simulink model "AEB_RuleBased_decisionmaking"  (R2021b)
settings: Solver=ode4  StartTime=0.0  StopTime=20  FixedStep=simtime  RelTol=1e-3
InitFcn:
  | clear all
  | 
  | % These are the starting values
  | initial_stopping_distance = 350; % set the stopping distance in m (6.368 and 11 is max deccel -9.5)
  | initial_velocity = 37.77; % set the initial velocity in m/s
  | road_grade = 0; %set road grade in degrees
  | sampletime = 0.01; %set the sample time of the controller
  | Ts = sampletime;
  | simtime = sampletime; %simulation set
  | 
  | initialdeccelcalc = -(initial_velocity^2)/(2*initial_stopping_distance);
libraries: simulink x2, sim3dlib x2, vdynlib x2, sim3dprobsensorlib x1, dspvision x1, autolibshared x1
settings Model: Creator=Tanmay Panchal  LastModifiedBy=tapan
settings SolverCC: AlgebraicLoopSolver=TrustRegion
settings DebuggingCC: SFMachineParentedDataDiag=warning

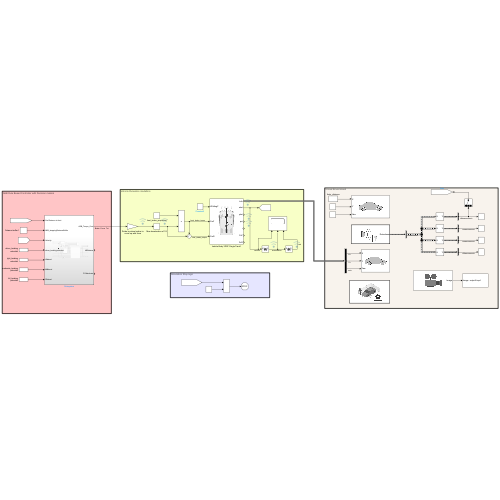
[thumbnail: Simulink's stored preview of the top-level diagram]
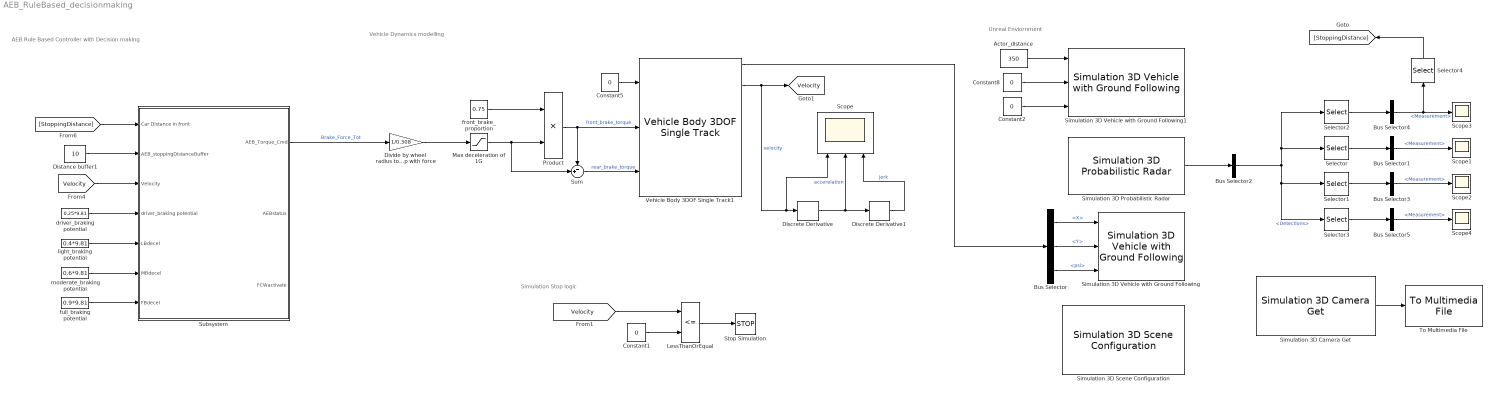
== system AEB_RuleBased_decisionmaking ==
  note: AEB Rule Based Controller with Decision making
  note: Vehicle Dynamics modelling
  note: Unreal Enviornment
  note: Simulation Stop logic
  Actor_distance : Constant  Value=350
  Bus Selector : BusSelector  OutputSignals=InertFrm.Cg.Disp.X,InertFrm.Cg.Disp.Y,InertFrm.Cg.Ang.psi
  Bus Selector{1,3..5} (4 alike) : BusSelector  OutputSignals=Measurement
  Bus Selector2 : BusSelector  OutputSignals=Detections
  Constant{1..2,5,8} (4 alike) : Constant  Value=0
  Discrete Derivative : simulink/Discrete/Discrete Derivative  gainval=1.0  ICPrevScaledInput=initial_velocity/sampletime  OutMin=[]  OutMax=[]  OutDataType=fixdt(1, 16)  OutScaling=2^-10  DoSatur=off
  Discrete Derivative1 : simulink/Discrete/Discrete Derivative  gainval=1.0  ICPrevScaledInput=0.0  OutMin=[]  OutMax=[]  OutDataType=fixdt(1, 16)  OutScaling=2^-10  DoSatur=off
  Distance buffer1 : Constant  Value=10
  Divide by wheel radius to come up with force : Gain  Gain=1/0.308
  LessThanOrEqual : RelationalOperator  Operator=<=  OutDataTypeStr=boolean  RndMeth=Simplest
  Max deceleration of 1G : Saturate  UpperLimit=0  LowerLimit=-1605*10
  Product : Product
  Scope : Scope  NumInputPorts=3
  Scope{1..4} (4 alike) : Scope
  Selector : Selector  InputPortWidth=10  IndexOptions=Index vector (dialog)  Indices=[3]  OutputSizes=1
  Selector1 : Selector  InputPortWidth=10  IndexOptions=Index vector (dialog)  Indices=[5]  OutputSizes=1
  Selector2 : Selector  InputPortWidth=10  IndexOptions=Index vector (dialog)  Indices=[1]  OutputSizes=1
  Selector3 : Selector  InputPortWidth=10  IndexOptions=Index vector (dialog)  Indices=[7]  OutputSizes=1
  Selector4 : Selector  InputPortWidth=3  IndexOptions=Index vector (dialog)  Indices=[1]  OutputSizes=1
  Simulation 3D Camera Get : sim3dlib/Simulation 3D Camera Get  Priority=1  sensorTag=Sim3dSensor3  sensorId=3  sensorName=Sim3dSensor3  vehTagList={'EGOVehicle';'Scene Origin';'Stray'}  vehTag=EGOVehicle  mountLoc=Rearview mirror  offsetFlag=off  tmountOffset=[0, 0, 0]  rmountOffset=[0, 0, 0]  HorizontalResolution=1280  VerticalResolution=720  HorizontalFOV=60  SampleTime=-1  mountPoint=[0.389999985694885 0 1.53999996185303]  mountOrientation=[0 0 0]  aMode=2  ID=3
      settings: SourceProductBaseCode=AE,DR,UV,VE
  Simulation 3D Probabilistic Radar : sim3dprobsensorlib/Simulation 3D Probabilistic Radar  Priority=1  sensorTag=Sim3dSensor1  sensorId=1  sensorName=Sim3dSensor1  vehTagList={'EGOVehicle';'Scene Origin';'Stray'}  vehTag=EGOVehicle  mountLoc=Origin  offsetFlag=off  tmountOffset=[0, 0, 0]  rmountOffset=[0, 0, 0]  AzimuthResolution=4  ElevationResolution=10  RangeResolution=2.5  RangeRateResolution=0.5  AzimuthBiasFraction=0.1  ElevationBiasFraction=0.1  RangeBiasFraction=0.05  RangeRateBiasFraction=0.05  FieldOfView=[ 20, 5 ]  DetectionRange=[ 1, 300 ]  RangeRateLimits=[ -100, 100 ]  DetectionProbability=0.9  FalseAlarmRate=1e-6  ReferenceRange=1000  ReferenceRCS=0  HasElevation=on  HasRangeRate=off  HasNoise=off  HasFalseAlarms=off  InitialSeedSource=Repeatable  InitialSeed=0  MaxNumDetections=10  DetectionCoordinates=Sensor Cartesian  SpecifyOutputBusName=off  BusName=BusSimulation3DRadarTruthSensor  SampleTime=-1  mountPoint=[0 0 0]  mountOrientation=[0 0 0]  aMode=3  ID=1
      settings: SourceProductBaseCode=AE,DR,UV,VE
  Simulation 3D Scene Configuration : sim3dlib/Simulation 3D Scene Configuration  Priority=0  ProjectFormat_internal=Default Scenes  ProjectFormat=Default Scenes  SceneDesc=Straight road  ProjectName=C:\Program Files\MATLAB\R2021b\toolbox\shared\sim3d_projects\automotive_project\UE4\WindowsNoEditor\VehicleSimulation.exe  ScenePath=/Game/Maps/HwStrght  vehTagList={'EGOVehicle';'Scene Origin';'Stray'}  vehTag=EGOVehicle  OpVisEn=off  Ts=0.01  EnableWindow=on  EnableWeather=off  SunAltitude=40.0  SunAzimuth=90  clouds=10  wind=1  fog=0  rain=0  sensorTag=MainCamera1  sensorId=1  sensorName=MainCamera1  mountLoc=Origin  offsetFlag=off  tmountOffset=[0, 0, 0]  rmountOffset=[0, 0, 0]  HorizontalResolution=1280  VerticalResolution=720  HorizontalFOV=60  mountPoint=[0 0 0]  mountOrientation=[0 0 0]  aMode=3  ID=1
      settings: SourceProductBaseCode=AE,DR,UV,VE
  Simulation 3D Vehicle with Ground Following : vdynlib/Vehicle Scenarios/Sim3D/Sim3D Vehicle/Components/Simulation 3D Vehicle with Ground Following  Priority=-1  PassVehMesh=Sport utility vehicle  PassVehMesh_Internal=Sport utility vehicle  MeshPath=/MathWorksSimulation/Vehicles/Muscle/Meshes/SK_MuscleCar.SK_MuscleCar  TrackWidth=1.9  WheelBase=3  WheelRadius=0.35  VehColor=Silver  VehColor_Internal=Silver  InitialPos=[0, 0, 0]  InitialRot=[0, 0, 0]  ActorName=EGOVehicle  VehLightsControl=off  HeadlightColor=[ 1, 1, 1 ]  HighBeamIntensity=100000  LowBeamIntensity=60000  HighBeamConeAngle=1.22  LowBeamConeAngle=1.22  LeftHeadlightOrientation=[ 0, 0 ]  RightHeadlightOrientation=[ 0, 0 ]  BrakelightIntensity=200  ReverselightIntensity=500  SignallightIntensity=500  SignallightPeriod=1  SignalPulseWidth=50  SampleTime=-1  ActorType=SimulinkVehicle  ID=C  aMode=2  ActorTag=EGOVehicle  CoordinateScheme=SAE
      settings: SourceProductBaseCode=VE
  Simulation 3D Vehicle with Ground Following1 : vdynlib/Vehicle Scenarios/Sim3D/Sim3D Vehicle/Components/Simulation 3D Vehicle with Ground Following  Priority=-1  PassVehMesh=Muscle car  PassVehMesh_Internal=Muscle car  MeshPath=/MathWorksSimulation/Vehicles/Muscle/Meshes/SK_MuscleCar.SK_MuscleCar  TrackWidth=1.9  WheelBase=3  WheelRadius=0.35  VehColor=Yellow  VehColor_Internal=Yellow  InitialPos=[0, 5, 0]  InitialRot=[0, 0, 0]  ActorName=Stray  VehLightsControl=off  HeadlightColor=[ 1, 1, 1 ]  HighBeamIntensity=100000  LowBeamIntensity=60000  HighBeamConeAngle=1.22  LowBeamConeAngle=1.22  LeftHeadlightOrientation=[ 0, 0 ]  RightHeadlightOrientation=[ 0, 0 ]  BrakelightIntensity=200  ReverselightIntensity=500  SignallightIntensity=500  SignallightPeriod=1  SignalPulseWidth=50  SampleTime=-1  ActorType=SimulinkVehicle  ID=C  aMode=2  ActorTag=Stray  CoordinateScheme=SAE
      settings: SourceProductBaseCode=VE
  Stop Simulation : Stop
  Subsystem : Subsystem
  Sum : Sum  Inputs=-+|
  To Multimedia File : dspvision/To Multimedia File  outputFilename=C:\Users\tapan\Desktop\output2.mp4  streamSelection=Video only  videoCompressor=None (uncompressed)  audioCompressor=None (uncompressed)  imagePorts=One multidimensional signal  fileType=MPEG4  audioDatatype=Determine from input data type  fourcc=RGB  videoQuality=75  mj2000CompFactor=10
  Vehicle Body 3DOF Single Track1 : autolibshared/Vehicle Body 3DOF Single Track  trackMode=Single (bicycle)  inputMode=External longitudinal forces  frontSteerMode=on  rearSteerMode=off  windMode=off  muMode=off  extFMode=off  extMMode=off  htchFMode=off  htchMMode=off  extXo=off  extpsio=off  extxdoto=off  extro=off  extYo=off  extTamb=off  extydoto=off  aMode=2  NF=2  NR=2  m=1625  a=1.135  b=1.465  h=0.509  dh=1  hh=0.2  X_o=0  xdot_o=initial_velocity  CalphaMode=off  sigmaMode=on  d=0  hl=0  w=[1.4,1.4]  Cy_f=12e3  Cy_r=11e3  sigma_f=.1  sigma_r=.1  alpha_f_brk=[-.1 .1]  Cy_f_data=[-9e3 9e3]  alpha_r_brk=[-.1 .1]  Cy_r_data=[-9e3 9e3]  Y_o=0  ydot_o=0  Izz=2045  psi_o=0  r_o=0  Af=2  Cd=.3  Cl=.1  Cpm=.1  beta_w=[0:0.01:0.3]  Cs=[0:0.03:0.9]  Cym=[0:0.01:0.3]  Pabs=101325  Tair=273  g=9.81  mu=1  xdot_tol=.01  Fznom=5000  Fxtire_sat=7e4  Fytire_sat=7e4  longOff=0  latOff=0  vertOff=0  wrapAng=off
      settings: SourceProductBaseCode=PW,DR,MT,UV,VE
  driver_braking potential : Constant  Value=0.25*9.81  SampleTime=-1
  front_brake_proportion : Constant  Value=0.75
  full_braking potential : Constant  Value=0.9*9.81  SampleTime=-1
  light_braking potential : Constant  Value=0.4*9.81  SampleTime=-1
  moderate_braking potential : Constant  Value=0.6*9.81  SampleTime=-1
  tag scope: Velocity=global
  wires:
  Discrete Derivative/1 -> Discrete Derivative1/1, Scope/2  "accerelation"
  Vehicle Body 3DOF Single Track1/2 -> Scope/1, Discrete Derivative/1, [Velocity]  "velocity"
  Discrete Derivative1/1 -> Scope/3  "jerk"
  LessThanOrEqual/1 -> Stop Simulation/1
  [Velocity] -> LessThanOrEqual/1
  Constant5/1 -> Vehicle Body 3DOF Single Track1/1
  Divide by wheel radius to come up with force/1 -> Max deceleration of 1G/1
  Max deceleration of 1G/1 -> Sum/2, Product/2
  Sum/1 -> Vehicle Body 3DOF Single Track1/3  "rear_brake_torque"
  front_brake_proportion/1 -> Product/1
  Product/1 -> Sum/1, Vehicle Body 3DOF Single Track1/2  "front_brake_torque"
  Bus Selector/2 -> Simulation 3D Vehicle with Ground Following/2  "<Y>"
  Bus Selector/1 -> Simulation 3D Vehicle with Ground Following/1  "<X>"
  Bus Selector/3 -> Simulation 3D Vehicle with Ground Following/3  "<psi>"
  Vehicle Body 3DOF Single Track1/1 -> Bus Selector/1
  Constant2/1 -> Simulation 3D Vehicle with Ground Following1/3
  Constant8/1 -> Simulation 3D Vehicle with Ground Following1/2
  Actor_distance/1 -> Simulation 3D Vehicle with Ground Following1/1
  Simulation 3D Probabilistic Radar/1 -> Bus Selector2/1
  Bus Selector2/1 -> Selector/1, Selector2/1, Selector3/1, Selector1/1  "<Detections>"
  Selector/1 -> Bus Selector1/1
  Bus Selector1/1 -> Scope1/1  "<Measurement>"
  Bus Selector3/1 -> Scope2/1  "<Measurement>"
  Selector1/1 -> Bus Selector3/1
  Selector2/1 -> Bus Selector4/1
  Bus Selector4/1 -> Scope3/1, Selector4/1  "<Measurement>"
  Bus Selector5/1 -> Scope4/1  "<Measurement>"
  Selector3/1 -> Bus Selector5/1
  Selector4/1 -> [StoppingDistance]
  Simulation 3D Camera Get/1 -> To Multimedia File/1
  Subsystem/1(AEB_Torque_Cmd) -> Divide by wheel radius to come up with force/1  "Brake_Force_Tot"
  Constant1/1 -> LessThanOrEqual/2
  [StoppingDistance] -> Subsystem/1(Car Distance in front)
  Distance buffer1/1 -> Subsystem/2(AEB_stoppingDistanceBuffer)
  [Velocity] -> Subsystem/3(Velocity)
  driver_braking potential/1 -> Subsystem/4(driver_braking potential)
  light_braking potential/1 -> Subsystem/5(LBdecel)
  moderate_braking potential/1 -> Subsystem/6(MBdecel)
  full_braking potential/1 -> Subsystem/7(FBdecel)

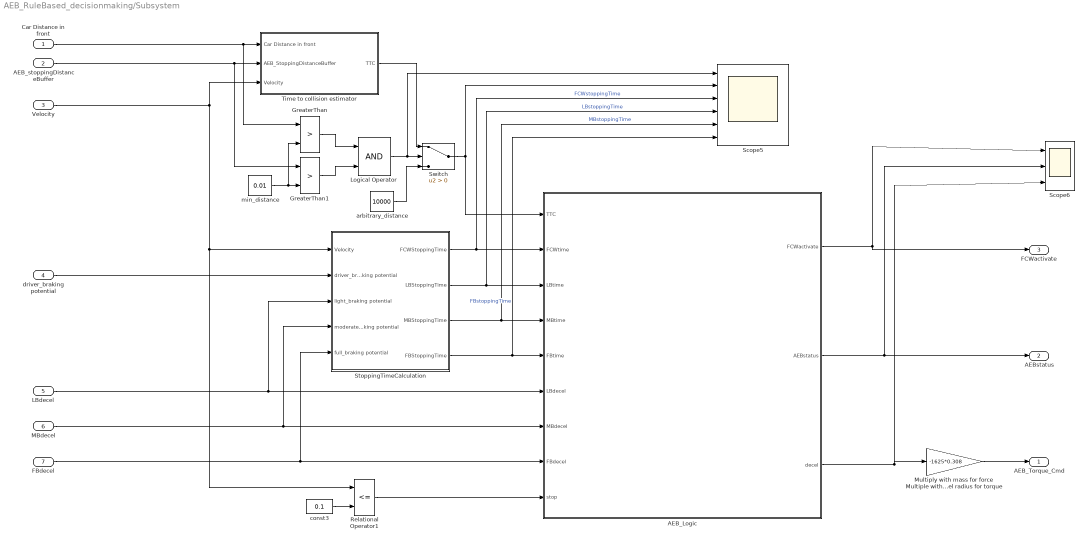
== system AEB_RuleBased_decisionmaking/Subsystem ==
  Car Distance in front : Inport
  AEB_stoppingDistanceBuffer : Inport  Port=2
  Velocity : Inport  Port=3
  driver_braking potential : Inport  Port=4
  LBdecel : Inport  Port=5
  MBdecel : Inport  Port=6
  FBdecel : Inport  Port=7
  AEB_Logic : Stateflow chart  TreatAsAtomicUnit=on
  GreaterThan : RelationalOperator  Operator=>  OutDataTypeStr=boolean  RndMeth=Simplest
  GreaterThan1 : RelationalOperator  Operator=>  OutDataTypeStr=boolean  RndMeth=Simplest
  Logical Operator : Logic  IconShape=distinctive  AllPortsSameDT=off  OutDataTypeStr=boolean
  Multiply with mass for force Multiple with wheel radius for torque : Gain  Gain=-1625*0.308
  Relational Operator1 : RelationalOperator  Operator=<=  OutDataTypeStr=boolean  RndMeth=Simplest
  Scope5 : Scope  NumInputPorts=6
  Scope6 : Scope  NumInputPorts=3
  StoppingTimeCalculation : Subsystem
  Switch : Switch  Criteria=u2 > Threshold
  Time to collision estimator : Subsystem
  arbitrary_distance : Constant  Value=10000
  const3 : Constant  Value=0.1  SampleTime=-1
  min_distance : Constant  Value=0.01
  AEB_Torque_Cmd : Outport
  AEBstatus : Outport  Port=2
  FCWactivate : Outport  Port=3
  wires:
  const3/1 -> Relational Operator1/2
  Velocity/1 -> Relational Operator1/1, StoppingTimeCalculation/1(Velocity), Time to collision estimator/3(Velocity)
  LBdecel/1 -> StoppingTimeCalculation/3(light_braking potential), AEB_Logic/6(LBdecel)
  AEB_Logic/2(AEBstatus) -> AEBstatus/1, Scope6/2
  StoppingTimeCalculation/4(FBStoppingTime) -> Scope5/6, AEB_Logic/5(FBtime)  "FBstoppingTime"
  FBdecel/1 -> StoppingTimeCalculation/5(full_braking potential), AEB_Logic/8(FBdecel)
  min_distance/1 -> GreaterThan/2, GreaterThan1/2
  AEB_stoppingDistanceBuffer/1 -> Time to collision estimator/2(AEB_StoppingDistanceBuffer), GreaterThan1/1
  Logical Operator/1 -> Scope5/1, Switch/2
  Relational Operator1/1 -> AEB_Logic/9(stop)
  StoppingTimeCalculation/2(LBStoppingTime) -> Scope5/4, AEB_Logic/3(LBtime)  "LBstoppingTime"
  driver_braking potential/1 -> StoppingTimeCalculation/2(driver_braking potential)
  AEB_Logic/3(decel) -> Multiply with mass for force Multiple with wheel radius for torque/1, Scope6/3
  MBdecel/1 -> StoppingTimeCalculation/4(moderate_braking potential), AEB_Logic/7(MBdecel)
  StoppingTimeCalculation/3(MBStoppingTime) -> Scope5/5, AEB_Logic/4(MBtime)  "MBstoppingTime"
  StoppingTimeCalculation/1(FCWStoppingTime) -> Scope5/3, AEB_Logic/2(FCWtime)  "FCWstoppingTime"
  Switch/1 -> Scope5/2, AEB_Logic/1(TTC)
  GreaterThan1/1 -> Logical Operator/2
  GreaterThan/1 -> Logical Operator/1
  Car Distance in front/1 -> Time to collision estimator/1(Car Distance in front), GreaterThan/1
  arbitrary_distance/1 -> Switch/3
  Time to collision estimator/1(TTC) -> Switch/1
  AEB_Logic/1(FCWactivate) -> FCWactivate/1, Scope6/1
  Multiply with mass for force Multiple with wheel radius for torque/1 -> AEB_Torque_Cmd/1

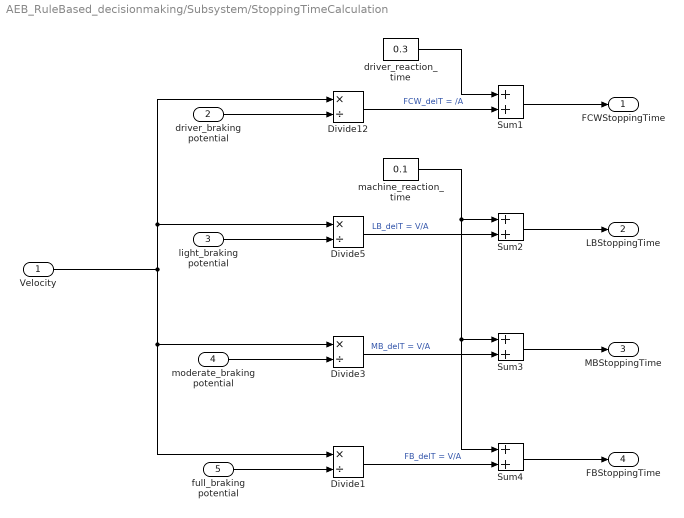
== system AEB_RuleBased_decisionmaking/Subsystem/StoppingTimeCalculation ==
  Velocity : Inport
  driver_braking potential : Inport  Port=2
  light_braking potential : Inport  Port=3
  moderate_braking potential : Inport  Port=4
  full_braking potential : Inport  Port=5
  Divide{1,3,5,12} (4 alike) : Product  Inputs=*/
  Sum{1..4} (4 alike) : Sum
  driver_reaction_time : Constant  Value=0.3  SampleTime=-1
  machine_reaction_time : Constant  Value=0.1  SampleTime=-1
  FCWStoppingTime : Outport  VectorParamsAs1DForOutWhenUnconnected=off
  LBStoppingTime : Outport  Port=2  VectorParamsAs1DForOutWhenUnconnected=off
  MBStoppingTime : Outport  Port=3  VectorParamsAs1DForOutWhenUnconnected=off
  FBStoppingTime : Outport  Port=4  VectorParamsAs1DForOutWhenUnconnected=off
  wires:
  Sum1/1 -> FCWStoppingTime/1
  Sum2/1 -> LBStoppingTime/1
  Sum3/1 -> MBStoppingTime/1
  Sum4/1 -> FBStoppingTime/1
  machine_reaction_time/1 -> Sum2/1, Sum3/1, Sum4/1
  Velocity/1 -> Divide12/1, Divide5/1, Divide3/1, Divide1/1
  Divide5/1 -> Sum2/2  "LB_delT = V/A"
  Divide3/1 -> Sum3/2  "MB_delT = V/A"
  Divide1/1 -> Sum4/2  "FB_delT = V/A"
  driver_reaction_time/1 -> Sum1/1
  Divide12/1 -> Sum1/2  "FCW_delT = /A"
  driver_braking potential/1 -> Divide12/2
  light_braking potential/1 -> Divide5/2
  moderate_braking potential/1 -> Divide3/2
  full_braking potential/1 -> Divide1/2

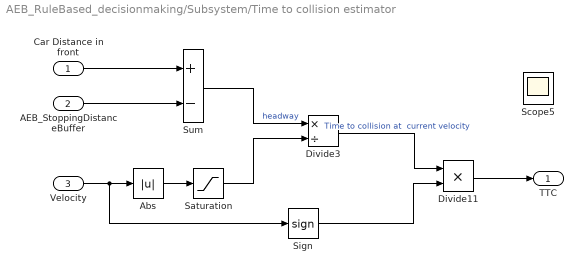
== system AEB_RuleBased_decisionmaking/Subsystem/Time to collision estimator ==
  Car Distance in front : Inport
  AEB_StoppingDistanceBuffer : Inport  Port=2
  Velocity : Inport  Port=3
  Abs : Abs
  Divide11 : Product  Inputs=**
  Divide3 : Product  Inputs=*/
  Saturation : Saturate  UpperLimit=400  LowerLimit=0.01
  Scope5 : Scope
  Sign : Signum
  Sum : Sum  Inputs=+-
  TTC : Outport  VectorParamsAs1DForOutWhenUnconnected=off
  wires:
  Velocity/1 -> Sign/1, Abs/1
  Car Distance in front/1 -> Sum/1
  Divide3/1 -> Divide11/1  "Time to collision at  current velocity"
  AEB_StoppingDistanceBuffer/1 -> Sum/2
  Sum/1 -> Divide3/1  "headway"
  Abs/1 -> Saturation/1
  Saturation/1 -> Divide3/2
  Sign/1 -> Divide11/2
  Divide11/1 -> TTC/1

== stateflow chart AEB_RuleBased_decisionmaking/Subsystem/AEB_Logic ==
  note: FCW/AEB Logic
  state Default
    entry: AEBstatus = 0;
    FCWactivate = 0;
    decel = 0;
  state FCW
    entry: AEBstatus = 0;
    FCWactivate = 1;
    decel = 0;
  state Light_braking
    entry: AEBstatus = 1;
    FCWactivate = 1;
    decel = LBdecel;
  state Full_Braking
    entry: AEBstatus = 3;
    FCWactivate = 1;
    decel = FBdecel;
  state Moderate_Braking
    entry: AEBstatus = 2;
    FCWactivate = 1;
    decel = MBdecel;
  (default) -> Default
  Moderate_Braking -> Default [order 3] : [stop==1]
  Full_Braking -> Default [order 2] : [stop==1]
  Light_braking -> Default [order 3] : [stop==1]
  Default -> FCW : [(abs(TTC)<=FCWtime)]
  FCW -> Default [order 2] : [abs(TTC)>1.2*FCWtime]
  Light_braking -> FCW [order 1] : [abs(TTC)>1.1*LBtime]
  FCW -> Light_braking [order 1] : [(abs(TTC) <= LBtime)]
  Moderate_Braking -> Light_braking [order 2] : [abs(TTC)>1.1*MBtime]
  Light_braking -> Moderate_Braking [order 2] : [(abs(TTC) <= MBtime)]
  Full_Braking -> Moderate_Braking [order 1] : [abs(TTC)>1.1*FBtime]
  Moderate_Braking -> Full_Braking [order 1] : [(abs(TTC) <= FBtime)]
  data: FCWactivate output; TTC input; FCWtime input; LBtime input; MBtime input; FBtime input; LBdecel input; MBdecel input; FBdecel input; AEBstatus output; decel output; stop input
